simulink model "sim_unitary_step"  (R2025b)
settings: Solver=VariableStepAuto  StartTime=0.0  StopTime=Tend  MaxStep=Ts*0.001  MinStep=Ts*0.0001  RelTol=1e-3
undefined symbols (not defined in the file): Ts
libraries: cstblocks x2
settings Model: Creator=davidecovolo  LastModifiedBy=davidecovolo

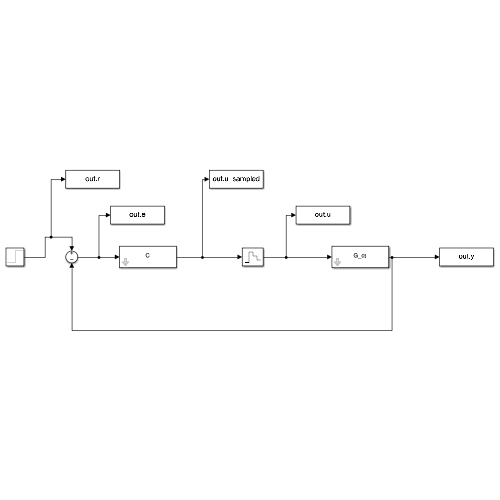
[thumbnail: Simulink's stored preview of the top-level diagram]
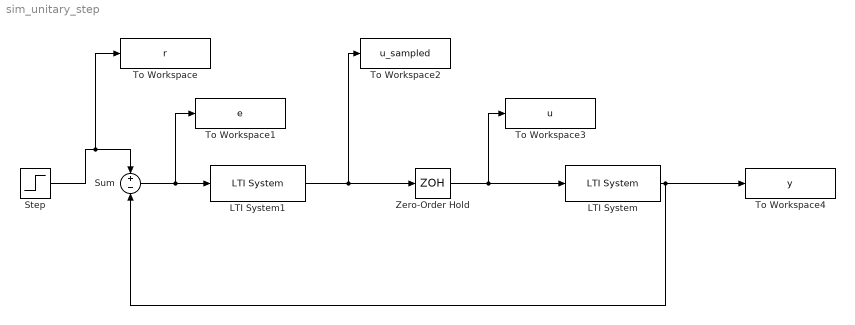
== system sim_unitary_step ==
  LTI System : cstblocks/LTI System  sys=G_ct  IC=[]  PadeOrder=0
  LTI System1 : cstblocks/LTI System  sys=C  IC=[]  PadeOrder=0
  Step : Step  Time=0  SampleTime=0
  Sum : Sum  Inputs=+-
  To Workspace : ToWorkspace  VariableName=r  SaveFormat=Timeseries  SampleTime=Ts*0.001
  To Workspace1 : ToWorkspace  VariableName=e  SaveFormat=Timeseries  SampleTime=Ts*0.001
  To Workspace2 : ToWorkspace  VariableName=u_sampled  SaveFormat=Timeseries  SampleTime=Ts
  To Workspace3 : ToWorkspace  VariableName=u  SaveFormat=Timeseries  SampleTime=Ts*0.001
  To Workspace4 : ToWorkspace  VariableName=y  SaveFormat=Timeseries  SampleTime=Ts*0.001
  Zero-Order Hold : ZeroOrderHold  SampleTime=Ts
  wires:
  Sum/1 -> To Workspace1/1, LTI System1/1
  LTI System1/1 -> To Workspace2/1, Zero-Order Hold/1
  Zero-Order Hold/1 -> To Workspace3/1, LTI System/1
  Step/1 -> To Workspace/1, Sum/1
  LTI System/1 -> Sum/2, To Workspace4/1
